simulink model "PD"  (R2019a)
settings: Solver=VariableStepAuto  StartTime=0.0  StopTime=10.0  RelTol=1e-3
undefined symbols (not defined in the file): Kd, Kp, parameter, x_com0, x_com_D, x_endEff0, x_endEff_D
settings Model: Creator=giga4  LastModifiedBy=pierluigi.amato

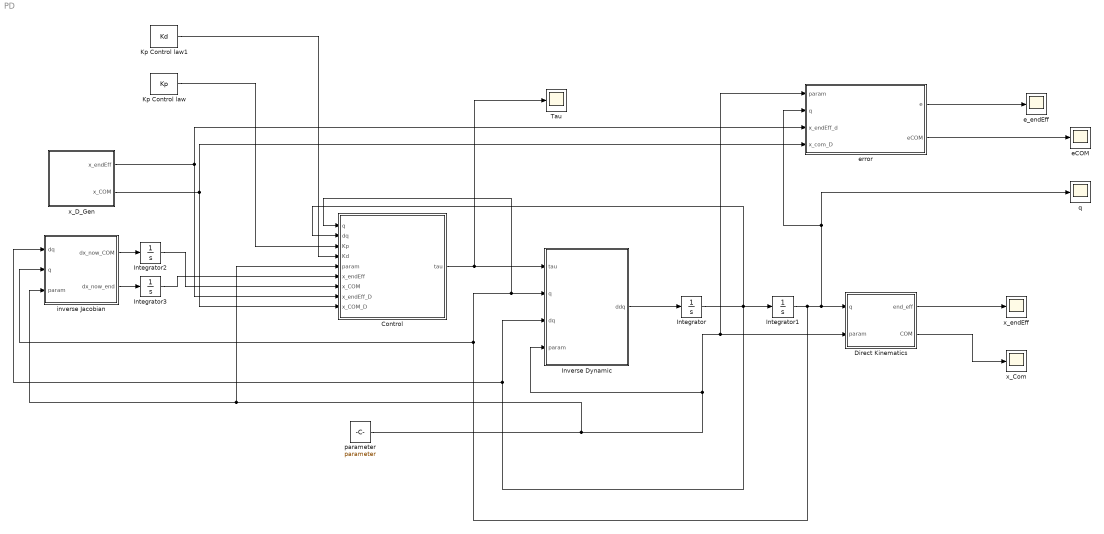
== system PD ==
  Control : MATLAB Function  TreatAsAtomicUnit=on
  "Direct Kinematics " : MATLAB Function  TreatAsAtomicUnit=on
  Integrator : Integrator  InitialCondition=[0,0,0,0,0,0]'
  Integrator1 : Integrator  InitialCondition=[0,0,0,0,0,0]'
  Integrator2 : Integrator  InitialCondition=x_com0
  Integrator3 : Integrator  InitialCondition=x_endEff0
  "Inverse Dynamic " : MATLAB Function  TreatAsAtomicUnit=on
  Kp Control law : Constant  Value=Kp
  Kp Control law1 : Constant  Value=Kd
  Tau : Scope
  eCOM : Scope
  e_endEff : Scope
  error : MATLAB Function  TreatAsAtomicUnit=on
  inverse Jacobian : MATLAB Function  TreatAsAtomicUnit=on
  "parameter " : Constant  Value=parameter
  q : Scope
  x_Com : Scope
  x_D_Gen : Subsystem
  x_endEff : Scope
  wires:
  "parameter "/1 -> Control/5(param), inverse Jacobian/3(param), "Inverse Dynamic "/4(param), error/1(param), "Direct Kinematics "/2(param)
  "Inverse Dynamic "/1(ddq) -> Integrator/1
  Integrator/1 -> inverse Jacobian/1(dq), "Inverse Dynamic "/3(dq), Control/2(dq), Integrator1/1
  Integrator1/1 -> inverse Jacobian/2(q), Control/1(q), "Inverse Dynamic "/2(q), error/2(q), q/1, "Direct Kinematics "/1(q)
  inverse Jacobian/1(dx_now_COM) -> Integrator2/1
  inverse Jacobian/2(dx_now_end) -> Integrator3/1
  Integrator3/1 -> Control/6(x_endEff)
  Kp Control law/1 -> Control/3(Kp)
  Control/1(tau) -> Tau/1, "Inverse Dynamic "/1(tau)
  Integrator2/1 -> Control/7(x_COM)
  "Direct Kinematics "/1(end_eff) -> x_endEff/1
  "Direct Kinematics "/2(COM) -> x_Com/1
  Kp Control law1/1 -> Control/4(Kd)
  error/1(e) -> e_endEff/1
  error/2(eCOM) -> eCOM/1
  x_D_Gen/1(x_endEff) -> error/3(x_endEff_d), Control/8(x_endEff_D)
  x_D_Gen/2(x_COM) -> error/4(x_com_D), Control/9(x_COM_D)

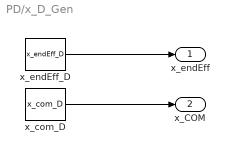
== system PD/x_D_Gen ==
  x_com_D : Constant  Value=x_com_D
  x_endEff_D : Constant  Value=x_endEff_D
  x_endEff : Outport
  x_COM : Outport  Port=2
  wires:
  x_endEff_D/1 -> x_endEff/1
  x_com_D/1 -> x_COM/1

== matlab function PD/Direct Kinematics  ==
  data: q input; end_eff output; param input; COM output
function [end_eff, COM] = DirectK(q,param)


    [Pcom, Etip,T00,T01,T12,T23,T34,T45,T56] =  forwardKinematics(param, q);
    
    
    end_eff = Etip(1:3,4);
    COM = Pcom;
    
end

== matlab function PD/Inverse Dynamic  ==
  data: tau input; q input; dq input; ddq output; param input
function ddq = inverseDynamic(tau,q,dq,param)

% B_f(q,param)
    B = B_f(q, param);
    G = G_f(q, param);
    C = C_f(q, dq, param);
    
    ddq = pinv(B)*(tau - G - C*dq);

end

== matlab function PD/inverse Jacobian ==
  data: dq input; q input; dx_now_COM output; param input; dx_now_end output
function [dx_now_COM,dx_now_end] = x_now(dq,q,param)

    dx_now_COM = JacobianCom(param, q)*dq;
    dx_now_end = JacobianEndEff(param, q)*dq;
end

== matlab function PD/Control ==
  data: q input; dq input; Kp input; Kd input; tau output; param input; x_endEff input; x_COM input; x_endEff_D input; x_COM_D input
function tau  = x_now(q, dq, Kp,Kd,param,x_endEff,x_COM, x_endEff_D, x_COM_D)
    
    J_endEff = JacobianEndEff(param, q)
    G = G_f(q,param);
    
    tau = J_endEff'*Kp*(x_endEff_D-x_endEff) - Kd*dq + G;
end

== matlab function PD/error ==
  data: param input; q input; e output; x_endEff_d input; x_com_D input; eCOM output
function [e,eCOM] = error(param, q, x_endEff_d, x_com_D)


    [Pcom, Etip,T00,T01,T12,T23,T34,T45,T56] =  forwardKinematics(param, q);
    x_endEff_now = Etip(1:3,4);
    x_COM = Pcom;
    
    e = x_endEff_d - x_endEff_now;
    eCOM = x_com_D - x_COM;

end
